simulink model "BD_SER_saber_cosim"  (Simulink 4.1.1)
settings: Solver=ode1  SolverMode=SingleTasking  StartTime=0.0  StopTime=max(cyc_mph(:,1))  FixedStep=1  MaxStep=1  RelTol=1e-3  AbsTol=1e-3
undefined symbols (not defined in the file): cs_fc_off2regen_pwr, cs_fc_spd_setpt_fun, cs_fc_trq_setpt_fun, cs_hi_soc, cs_lo_soc, cyc_mph, ess_max_volts_fun, ess_min_volts_fun, ess_on, ex_calc, fc_emis, fc_map_spd, fc_max_trq, fc_on, fc_spd_scale, fc_trq_scale, fd_ratio, gb_dnshift_load, gb_dnshift_spd, gb_gears_num, gb_num_init, gb_ratio, gb_shift_delay, gb_upshift_load, gb_upshift_spd, gc_map_spd, gc_max_trq, gc_spd_scale, gc_trq_scale, mc_map_spd, mc_max_trq, mc_spd_scale, mc_trq_scale, tc_gc_to_fc_ratio_fun, time_step, tx_speed_dep, vc_idle_bool, vc_idle_spd, wh_radius
libraries: lib_cosimulation x10, lib_outputs x8, lib_controls x5, lib_wheel x2, lib_help x2, lib_transmission x2, lib_accessory x2, lib_interactive x1, lib_drive_cycle x1, lib_exhaust x1, lib_fuel_converter x1, lib_vehicle x1
(part 1 of 2)
settings Model: LastModifiedBy=ssprik  SaveTime=off  SaveOutput=off  LimitDataPoints=off  UnconnectedLineMsg=none  RTWTemplateMakefile=grt_vc.tmf  ExtModeTrigMode=oneshot  ExtModeArmWhenConnect=off
settings Model: ModifiedComment=|
  | mokeefe -- Thu Apr 18 08:09:28 2002 -- Version 1.121
  | saving the model:
  | o "without the model browser open"
  | o with only top-level screen visible
  | o and with "fit to view" enabled
settings Model: ModifiedHistory=|
  | mokeefe -- Thu Apr 18 08:09:28 2002 -- Version 1.121
  | saving the model:
  | o "without the model browser open"
  | o with only top-level screen visible
  | o and with "fit to view" enabled

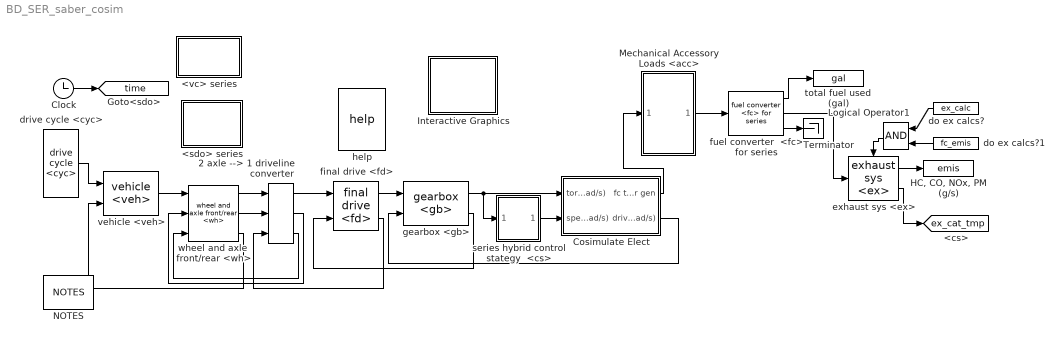
== system BD_SER_saber_cosim ==
  2 axle --> 1 driveline converter : lib_wheel/2 axle --> 1 driveline converter
      settings: RTWFcnNameOpts=Auto  RTWFileNameOpts=Auto
  <sdo> series : Subsystem
      settings: RTWFcnNameOpts=Auto  RTWFileNameOpts=Auto
      mask Display: image(imread('bdi_sdo.jpg'))
  <vc> series : Subsystem
      settings: RTWFcnNameOpts=Auto  RTWFileNameOpts=Auto
      mask Display: image(imread('bdi_vc.jpg'))
  Clock : Clock
      settings: DisplayTime=off  Decimation=10
  Cosimulate Elect : Subsystem  AncestorBlock=lib_cosimulation/SaberCosim
      settings: RTWFcnNameOpts=Auto  RTWFileNameOpts=Auto
      mask Display: image(imread('series_cosim.bmp'))
  "HC, CO, NOx, PM (g/s)" : ToWorkspace  VariableName=emis  SampleTime=0  SaveFormat=Array
  Interactive Graphics : Subsystem  BlockChoice=off
      link override off/Live Inputs/veh/roll res interactive: BlockChoice=roll res force req (N)
      settings: AttributesFormatString=%<BlockChoice>  TemplateBlock=lib_interactive/Interactive Graphics  MemberBlocks=off,on  RTWFcnNameOpts=Auto  RTWFileNameOpts=Auto
  Logical Operator1 : Logic  Orientation=left  Operator=AND  Inputs=2
  Mechanical Accessory Loads <acc> : Subsystem
      settings: RTWFcnNameOpts=Auto  RTWFileNameOpts=Auto
      mask Display: image(imread('bdi_acc_pic.bmp'))
  NOTES : lib_help/NOTES
  Terminator : Terminator
  do ex calcs? : Constant  Orientation=left  Value=ex_calc
  do ex calcs?1 : Constant  Orientation=left  Value=fc_emis
  drive cycle <cyc> : lib_drive_cycle/drive cycle <cyc>
  exhaust sys <ex> : lib_exhaust/exhaust sys <ex>
  final drive <fd> : lib_transmission/final drive <fd>
  fuel converter  <fc> for series : lib_fuel_converter/fuel converter  <fc> for series
      link override fuel use and EO emis Configurable Subsystem: BlockChoice=fuel use and EO emis
  gearbox <gb> : lib_transmission/gearbox <gb>
  help : lib_help/help
  series hybrid control stategy  <cs> : Subsystem
      settings: RTWFcnNameOpts=Auto  RTWFileNameOpts=Auto
      mask Display: image(imread('bdi_cs.jpg'))
  total fuel used  (gal) : ToWorkspace  VariableName=gal  SampleTime=0  SaveFormat=Array
  vehicle <veh> : lib_vehicle/vehicle <veh>
      link override config force req'd to overcome rolling resistance: BlockChoice=force req'd to overcome rolling resistance (N)
      link override config vehicle speed: BlockChoice=vehicle speed (m/s)
      link override rolling resistance force: BlockChoice=force req'd to overcome rolling resistance (N)
      link override vehicle speed: BlockChoice=vehicle speed (m/s)
  wheel and axle  front/rear <wh> : lib_wheel/wheel and axle  front//rear <wh>
  tag scope: ex_cat_tmp=global, time=global
  wires:
  gearbox <gb>/1 -> Cosimulate Elect/1(torque and speed req'd at input side of gearbox (Nm),(rad/s)), series hybrid control stategy  <cs>/1(gb trq & spd r)
  gearbox <gb>/2 -> final drive <fd>/2
  final drive <fd>/1 -> gearbox <gb>/1
  drive cycle <cyc>/1 -> vehicle <veh>/1
  Clock/1 -> [time]
  fuel converter  <fc> for series/2 -> exhaust sys <ex>/1
  fuel converter  <fc> for series/1 -> total fuel used  (gal)/1
  Logical Operator1/1 -> exhaust sys <ex>/Enable
  do ex calcs?/1 -> Logical Operator1/1
  exhaust sys <ex>/1 -> "HC, CO, NOx, PM (g/s)"/1
  do ex calcs?1/1 -> Logical Operator1/2
  exhaust sys <ex>/2 -> [ex_cat_tmp]
  Cosimulate Elect/2("drive torque and speed avail. at rotor (Nm), (rad/s)") -> gearbox <gb>/2
  series hybrid control stategy  <cs>/1(engine speed and torque (Nm) (rad/s)) -> Cosimulate Elect/2(speed and torque  avail from fc  (Nm) (rad/s))
  fuel converter  <fc> for series/3 -> Terminator/1
  Cosimulate Elect/1(fc trq and spd req'd for gen) -> Mechanical Accessory Loads <acc>/1(trq and spd)
  Mechanical Accessory Loads <acc>/1(trq and spd1) -> fuel converter  <fc> for series/1
  wheel and axle  front/rear <wh>/1 -> 2 axle --> 1 driveline converter/1
  wheel and axle  front/rear <wh>/2 -> 2 axle --> 1 driveline converter/2
  2 axle --> 1 driveline converter/1 -> final drive <fd>/1
  2 axle --> 1 driveline converter/2 -> wheel and axle  front/rear <wh>/2
  2 axle --> 1 driveline converter/3 -> wheel and axle  front/rear <wh>/3
  vehicle <veh>/1 -> wheel and axle  front/rear <wh>/1
  final drive <fd>/2 -> 2 axle --> 1 driveline converter/3
  wheel and axle  front/rear <wh>/3 -> vehicle <veh>/2

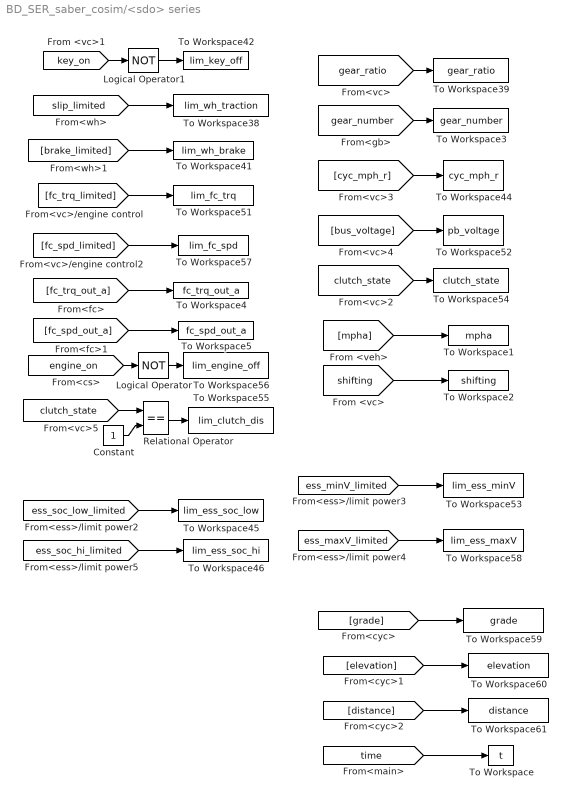
== system BD_SER_saber_cosim/<sdo> series ==
  Constant : Constant  Value=1
  Logical Operator : Logic  Operator=NOT  Inputs=1
  Logical Operator1 : Logic  Operator=NOT  Inputs=1
  Relational Operator : RelationalOperator  Operator===
  To Workspace : ToWorkspace  VariableName=t  SampleTime=0  SaveFormat=Array
  To Workspace1 : ToWorkspace  VariableName=mpha  SampleTime=-1  SaveFormat=Array
  To Workspace2 : ToWorkspace  VariableName=shifting  SampleTime=-1  SaveFormat=Array
  To Workspace3 : ToWorkspace  VariableName=gear_number  SampleTime=-1  SaveFormat=Array
  To Workspace38 : ToWorkspace  VariableName=lim_wh_traction  SampleTime=-1  SaveFormat=Array
  To Workspace39 : ToWorkspace  VariableName=gear_ratio  SampleTime=-1  SaveFormat=Array
  To Workspace4 : ToWorkspace  VariableName=fc_trq_out_a  SampleTime=-1  SaveFormat=Array
  To Workspace41 : ToWorkspace  VariableName=lim_wh_brake  SampleTime=-1  SaveFormat=Array
  To Workspace42 : ToWorkspace  VariableName=lim_key_off  SampleTime=-1  SaveFormat=Array
  To Workspace44 : ToWorkspace  VariableName=cyc_mph_r  SampleTime=-1  SaveFormat=Array
  To Workspace45 : ToWorkspace  VariableName=lim_ess_soc_low  SampleTime=-1  SaveFormat=Array
  To Workspace46 : ToWorkspace  VariableName=lim_ess_soc_hi  SampleTime=-1  SaveFormat=Array
  To Workspace5 : ToWorkspace  VariableName=fc_spd_out_a  SampleTime=-1  SaveFormat=Array
  To Workspace51 : ToWorkspace  VariableName=lim_fc_trq  SampleTime=-1  SaveFormat=Array
  To Workspace52 : ToWorkspace  VariableName=pb_voltage  SampleTime=-1  SaveFormat=Array
  To Workspace53 : ToWorkspace  VariableName=lim_ess_minV  SampleTime=-1  SaveFormat=Array
  To Workspace54 : ToWorkspace  VariableName=clutch_state  SampleTime=-1  SaveFormat=Array
  To Workspace55 : ToWorkspace  VariableName=lim_clutch_dis  SampleTime=-1  SaveFormat=Array
  To Workspace56 : ToWorkspace  VariableName=lim_engine_off  SampleTime=-1  SaveFormat=Array
  To Workspace57 : ToWorkspace  VariableName=lim_fc_spd  SampleTime=-1  SaveFormat=Array
  To Workspace58 : ToWorkspace  VariableName=lim_ess_maxV  SampleTime=-1  SaveFormat=Array
  To Workspace59 : ToWorkspace  VariableName=grade  SampleTime=-1  SaveFormat=Array
  To Workspace60 : ToWorkspace  VariableName=elevation  SampleTime=-1  SaveFormat=Array
  To Workspace61 : ToWorkspace  VariableName=distance  SampleTime=-1  SaveFormat=Array
  wires:
  [time] -> To Workspace/1
  [clutch_state] -> Relational Operator/1
  [fc_spd_out_a] -> To Workspace5/1
  [fc_trq_out_a] -> To Workspace4/1
  [ess_soc_hi_limited] -> To Workspace46/1
  [ess_soc_low_limited] -> To Workspace45/1
  Logical Operator/1 -> To Workspace56/1
  [engine_on] -> Logical Operator/1
  Constant/1 -> Relational Operator/2
  Relational Operator/1 -> To Workspace55/1
  [distance] -> To Workspace61/1
  [elevation] -> To Workspace60/1
  [grade] -> To Workspace59/1
  [ess_minV_limited] -> To Workspace53/1
  [ess_maxV_limited] -> To Workspace58/1
  Logical Operator1/1 -> To Workspace42/1
  [key_on] -> Logical Operator1/1
  [shifting] -> To Workspace2/1
  [mpha] -> To Workspace1/1
  [clutch_state] -> To Workspace54/1
  [bus_voltage] -> To Workspace52/1
  [cyc_mph_r] -> To Workspace44/1
  [gear_ratio] -> To Workspace39/1
  [slip_limited] -> To Workspace38/1
  [brake_limited] -> To Workspace41/1
  [fc_spd_limited] -> To Workspace57/1
  [fc_trq_limited] -> To Workspace51/1
  [gear_number] -> To Workspace3/1

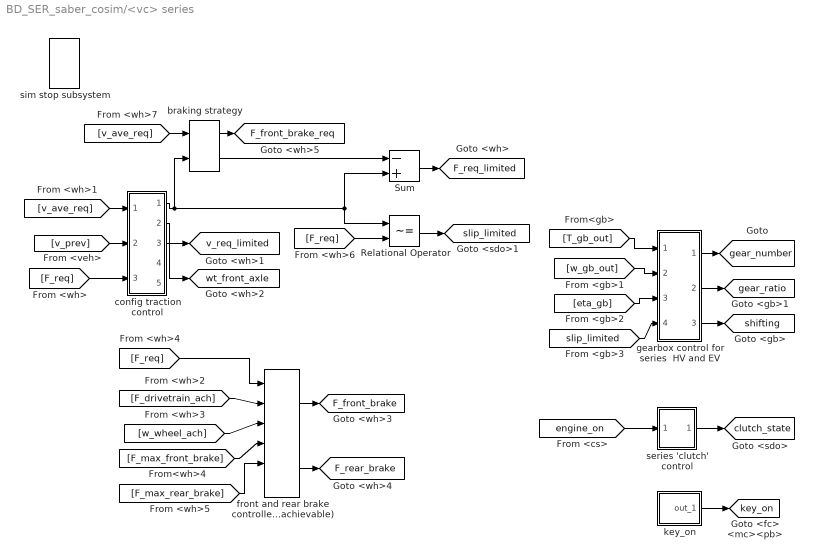
== system BD_SER_saber_cosim/<vc> series ==
  Relational Operator : RelationalOperator  Operator=~=
  Sum : Sum  Inputs=-+  SaturateOnIntegerOverflow=on
  braking strategy : lib_controls/SubSystem/braking strategy
      settings: RTWFcnNameOpts=Auto  RTWFileNameOpts=Auto
  config traction control : Subsystem  BlockChoice=traction control 2 axle
      settings: AttributesFormatString=%<BlockChoice>  TemplateBlock=lib_controls/SubSystem/config traction control  MemberBlocks=traction control 2 axle,traction control J2452 2 axle  RTWFcnNameOpts=Auto  RTWFileNameOpts=Auto
  front and rear brake controller (achievable) : lib_controls/SubSystem/front and rear brake controller (achievable)
      settings: RTWFcnNameOpts=Auto  RTWFileNameOpts=Auto
  gearbox control for series  HV and EV : Subsystem
      settings: RTWFcnNameOpts=Auto  RTWFileNameOpts=Auto
  key_on : Subsystem  mask(Repeating table){@1=vc_key_on(:,1), @2=vc_key_on(:,2)}
      mask prompts: @1 "Time values:"; @2 "Output values:"
      mask help:
      | Repeating table.
      | Enter values of time and output for first cycle.
      mask init:
      | period = max(@1); t = @1; y = @2;
      settings: RTWFcnNameOpts=Auto  RTWFileNameOpts=Auto
      mask Help: Repeats cycle given in table. Time values should be monotonically increasing.
  series 'clutch' control : Subsystem
      settings: RTWFcnNameOpts=Auto  RTWFileNameOpts=Auto
  sim stop subsystem : lib_controls/SubSystem/sim stop subsystem
      settings: RTWFcnNameOpts=Auto  RTWFileNameOpts=Auto
  tag scope: F_front_brake=global, F_front_brake_req=global, F_rear_brake=global, F_req_limited=global, clutch_state=global, gear_number=global, gear_ratio=global, key_on=global, shifting=global, slip_limited=global, v_req_limited=global, wt_front_axle=global
  wires:
  gearbox control for series  HV and EV/1("gear number, out") -> [gear_number]
  gearbox control for series  HV and EV/2("gear ratio, out") -> [gear_ratio]
  gearbox control for series  HV and EV/3("shifting, out") -> [shifting]
  [v_ave_req] -> config traction control/1(time-average vehicle speed  req'd (m/s))
  [F_req] -> Relational Operator/2
  Relational Operator/1 -> [slip_limited]
  Sum/1 -> [F_req_limited]
  [F_req] -> config traction control/3(total tractive force req'd (N))
  config traction control/3(weight on front axle (N)) -> [wt_front_axle]
  config traction control/2(req'd speed (m/s)) -> [v_req_limited]
  [v_prev] -> config traction control/2(vehicle speed at beginning of time  step (m/s))
  config traction control/1(req'd force (N)) -> Relational Operator/1, Sum/2, braking strategy/2
  braking strategy/2 -> Sum/1
  [v_ave_req] -> braking strategy/1
  braking strategy/1 -> [F_front_brake_req]
  [F_req] -> front and rear brake controller (achievable)/1
  front and rear brake controller (achievable)/2 -> [F_rear_brake]
  [F_max_rear_brake] -> front and rear brake controller (achievable)/5
  [F_max_front_brake] -> front and rear brake controller (achievable)/4
  [w_wheel_ach] -> front and rear brake controller (achievable)/3
  [F_drivetrain_ach] -> front and rear brake controller (achievable)/2
  front and rear brake controller (achievable)/1 -> [F_front_brake]
  key_on/1(out_1) -> [key_on]
  [engine_on] -> series 'clutch' control/1(engine on)
  series 'clutch' control/1(clutch state) -> [clutch_state]
  [slip_limited] -> gearbox control for series  HV and EV/4(tires are at traction limit)
  [T_gb_out] -> gearbox control for series  HV and EV/1(gb_trq_out_r)
  [w_gb_out] -> gearbox control for series  HV and EV/2(gb_spd_out_r)
  [eta_gb] -> gearbox control for series  HV and EV/3(prev. Pout/Pin)

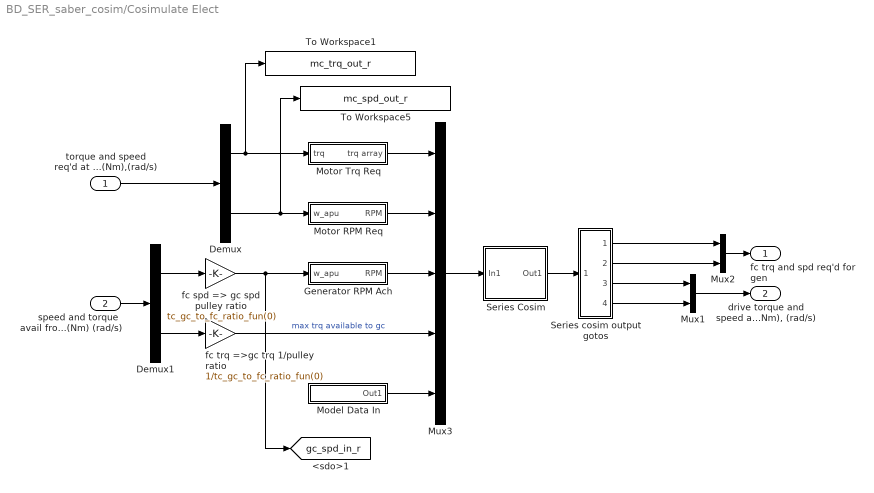
== system BD_SER_saber_cosim/Cosimulate Elect ==
  torque and speed req'd at input side of gearbox (Nm),(rad/s) : Inport  Port=1  LatchInput=off
  speed and torque  avail from fc  (Nm) (rad/s) : Inport  Port=2  LatchInput=off  PortDimensions=2
  Demux : Demux  Outputs=2  BusSelectionMode=off
  Demux1 : Demux  Outputs=2  BusSelectionMode=off
  Generator RPM Ach : Subsystem
      settings: RTWFcnNameOpts=Auto  RTWFileNameOpts=Auto
  Model Data In : Subsystem
      settings: RTWFcnNameOpts=Auto  RTWFileNameOpts=Auto
      mask Display: disp('Series')
  Motor RPM Req : Subsystem
      settings: RTWFcnNameOpts=Auto  RTWFileNameOpts=Auto
  Motor Trq Req : Subsystem
      settings: RTWFcnNameOpts=Auto  RTWFileNameOpts=Auto
  Mux1 : Mux  Inputs=2
  Mux2 : Mux  Inputs=2
  Mux3 : Mux  Inputs=5
  Series Cosim : Subsystem  BlockChoice=Saber Text File Exchange
      settings: AttributesFormatString=%<BlockChoice>  TemplateBlock=lib_cosimulation/Series Cosim  MemberBlocks=Saber Text File Exchange,Series Saber Cosim,Series Simplorer Cosim  RTWFcnNameOpts=Auto  RTWFileNameOpts=Auto
  Series cosim output gotos : Subsystem
      settings: RTWFcnNameOpts=Auto  RTWFileNameOpts=Auto
  To Workspace1 : ToWorkspace  VariableName=mc_trq_out_r  SampleTime=-1  SaveFormat=Array
  To Workspace5 : ToWorkspace  VariableName=mc_spd_out_r  SampleTime=-1  SaveFormat=Array
  fc spd => gc spd pulley ratio : Gain  Gain=tc_gc_to_fc_ratio_fun(0)  Multiplication=Element-wise(K.*u)  SaturateOnIntegerOverflow=on
  fc trq =>gc trq 1/pulley ratio : Gain  Gain=1/tc_gc_to_fc_ratio_fun(0)  Multiplication=Element-wise(K.*u)  SaturateOnIntegerOverflow=on
  fc trq and spd req'd for gen : Outport  Port=1
  "drive torque and speed avail. at rotor (Nm), (rad/s)" : Outport  Port=2  InitialOutput=0
  tag scope: gc_spd_in_r=global
  wires:
  torque and speed req'd at input side of gearbox (Nm),(rad/s)/1 -> Demux/1
  Mux3/1 -> Series Cosim/1(In1)
  Series Cosim/1(Out1) -> Series cosim output gotos/1(In1)
  Mux1/1 -> "drive torque and speed avail. at rotor (Nm), (rad/s)"/1
  Series cosim output gotos/1(fc_trq_r) -> Mux2/1
  Demux/2 -> Motor RPM Req/1(w_apu), To Workspace5/1
  Motor RPM Req/1(RPM) -> Mux3/2
  Demux/1 -> Motor Trq Req/1(trq), To Workspace1/1
  Motor Trq Req/1(trq array) -> Mux3/1
  Series cosim output gotos/4(mc_spd) -> Mux1/2
  Series cosim output gotos/3(mc_trq) -> Mux1/1
  Series cosim output gotos/2(fc_spd_r) -> Mux2/2
  Mux2/1 -> fc trq and spd req'd for gen/1
  Generator RPM Ach/1(RPM) -> Mux3/3
  fc spd => gc spd pulley ratio/1 -> Generator RPM Ach/1(w_apu), [gc_spd_in_r]
  Model Data In/1(Out1) -> Mux3/5
  Demux1/1 -> fc spd => gc spd pulley ratio/1
  Demux1/2 -> fc trq =>gc trq 1/pulley ratio/1
  speed and torque  avail from fc  (Nm) (rad/s)/1 -> Demux1/1
  fc trq =>gc trq 1/pulley ratio/1 -> Mux3/4  "max trq available to gc"

== system BD_SER_saber_cosim/Interactive Graphics ==
  off : lib_interactive/off  Tag=Altia_off  Orientation=up

== system BD_SER_saber_cosim/Mechanical Accessory Loads <acc> ==
  trq and spd : Inport  Port=1  LatchInput=off
  Demux2 : Demux  Outputs=2  BusSelectionMode=off
  Mux2 : Mux  Inputs=2
  Sum : Sum  Inputs=++  SaturateOnIntegerOverflow=on
  trq and spd1 : Outport  Port=1
  wires:
  Mux2/1 -> trq and spd1/1
  trq and spd/1 -> Demux2/1
  Sum/1 -> Mux2/1
  [acc_total_mech_trq] -> Sum/1
  Demux2/1 -> Sum/2
  Demux2/2 -> Mux2/2

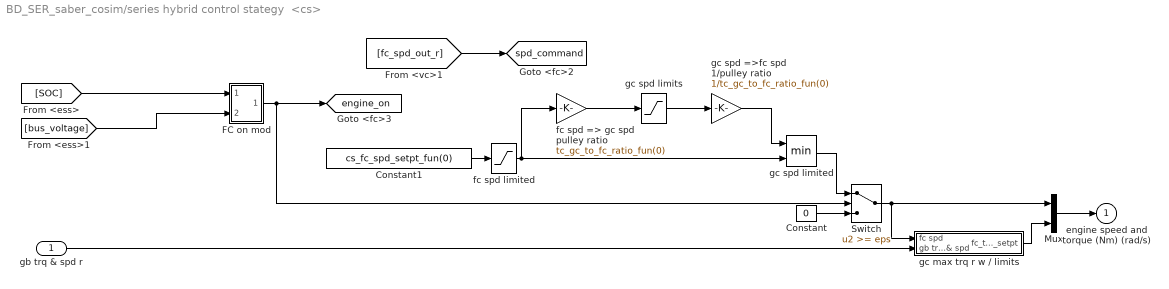
== system BD_SER_saber_cosim/series hybrid control stategy  <cs> ==
  gb trq & spd r : Inport  Port=1  LatchInput=off
  Constant : Constant  Value=0
  Constant1 : Constant  Value=cs_fc_spd_setpt_fun(0)
  FC on mod : Subsystem
      settings: RTWFcnNameOpts=Auto  RTWFileNameOpts=Auto
  Mux : Mux  Inputs=2
  Switch : Switch  Threshold=eps
  fc spd limited : Saturate  UpperLimit=max(fc_map_spd)*fc_spd_scale  LowerLimit=0  LinearizeAsGain=on
  fc spd => gc spd pulley ratio : Gain  Gain=tc_gc_to_fc_ratio_fun(0)  Multiplication=Element-wise(K.*u)  SaturateOnIntegerOverflow=on
  gc max trq r w / limits : Subsystem
      settings: RTWFcnNameOpts=Auto  RTWFileNameOpts=Auto
  gc spd limited : MinMax  Function=min  Inputs=2
  gc spd limits : Saturate  UpperLimit=max(gc_map_spd)*gc_spd_scale  LowerLimit=0  LinearizeAsGain=on
  gc spd =>fc spd 1/pulley ratio : Gain  Gain=1/tc_gc_to_fc_ratio_fun(0)  Multiplication=Element-wise(K.*u)  SaturateOnIntegerOverflow=on
  engine speed and torque (Nm) (rad/s) : Outport  Port=1  InitialOutput=0
  tag scope: engine_on=global, spd_command=global
  wires:
  FC on mod/1(FC on) -> Switch/2, [engine_on]
  [fc_spd_out_r] -> [spd_command]
  Constant/1 -> Switch/3
  gb trq & spd r/1 -> gc max trq r w / limits/2(gb trq & spd)
  [bus_voltage] -> FC on mod/2(bus voltage)
  [SOC] -> FC on mod/1(SOC)
  Constant1/1 -> fc spd limited/1
  fc spd limited/1 -> gc spd limited/2, fc spd => gc spd pulley ratio/1
  Mux/1 -> engine speed and torque (Nm) (rad/s)/1
  Switch/1 -> gc max trq r w / limits/1(fc spd), Mux/1
  gc max trq r w / limits/1(fc_trq_setpt) -> Mux/2
  gc spd limited/1 -> Switch/1
  fc spd => gc spd pulley ratio/1 -> gc spd limits/1
  gc spd =>fc spd 1/pulley ratio/1 -> gc spd limited/1
  gc spd limits/1 -> gc spd =>fc spd 1/pulley ratio/1

== system BD_SER_saber_cosim/<vc> series/config traction control ==
  time-average vehicle speed  req'd (m/s) : Inport  Port=1  LatchInput=off
  vehicle speed at beginning of time  step (m/s) : Inport  Port=2  LatchInput=off
  total tractive force req'd (N) : Inport  Port=3  LatchInput=off
  traction control 2 axle : lib_controls/SubSystem/traction control 2 axle
      settings: RTWFcnNameOpts=Auto  RTWFileNameOpts=Auto
  req'd force (N) : Outport  Port=1
  req'd speed (m/s) : Outport  Port=2
  weight on front axle (N) : Outport  Port=3
  weight on rear axle (N) : Outport  Port=4
  front/total  traction ratio : Outport  Port=5
  wires:
  time-average vehicle speed  req'd (m/s)/1 -> traction control 2 axle/1
  vehicle speed at beginning of time  step (m/s)/1 -> traction control 2 axle/2
  total tractive force req'd (N)/1 -> traction control 2 axle/3
  traction control 2 axle/1 -> req'd force (N)/1
  traction control 2 axle/2 -> req'd speed (m/s)/1
  traction control 2 axle/3 -> weight on front axle (N)/1
  traction control 2 axle/4 -> weight on rear axle (N)/1
  traction control 2 axle/5 -> front/total  traction ratio/1

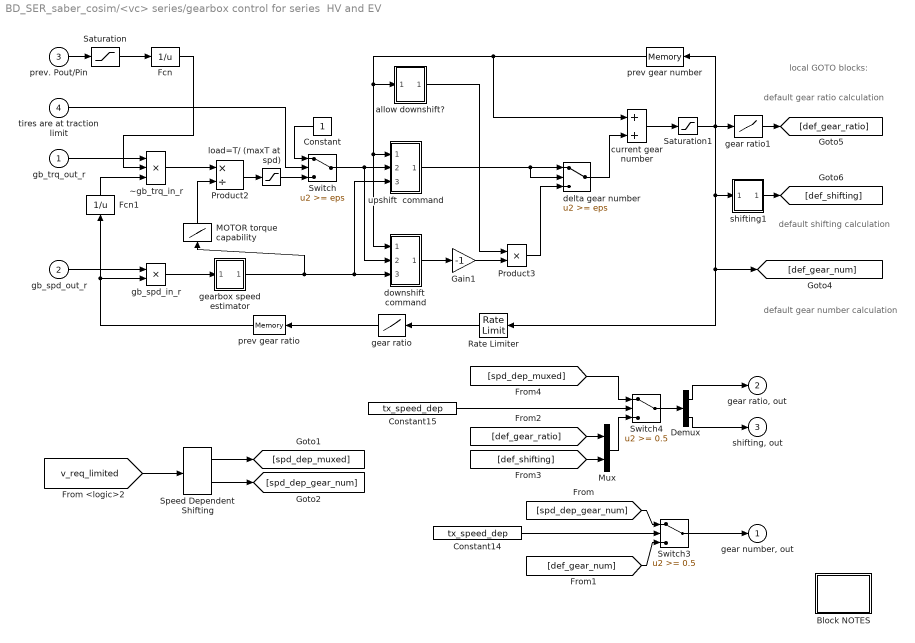
== system BD_SER_saber_cosim/<vc> series/gearbox control for series  HV and EV ==
  note: local GOTO blocks:
  note: default gear ratio
      | calculation
  note: default shifting
      | calculation
  note: default gear number
      | calculation
  gb_trq_out_r : Inport  Port=1  LatchInput=off
  gb_spd_out_r : Inport  Port=2  LatchInput=off
  prev. Pout/Pin : Inport  Port=3  LatchInput=off
  tires are at traction limit : Inport  Port=4  LatchInput=off
  Block NOTES : Subsystem
      settings: RTWFcnNameOpts=Auto  RTWFileNameOpts=Auto
      mask Display: disp('Block\nNOTES')
  Constant : Constant  Orientation=left  Value=1
  Constant14 : Constant  Value=tx_speed_dep
  Constant15 : Constant  Value=tx_speed_dep
  Demux : Demux  Outputs=2  BusSelectionMode=off
  Fcn : Fcn  Expr=1/u
  Fcn1 : Fcn  Orientation=up  Expr=1/u
  Gain1 : Gain  Gain=-1  Multiplication=Element-wise(K.*u)  SaturateOnIntegerOverflow=on
  MOTOR torque capability : Lookup  Orientation=up  InputValues=mc_map_spd*mc_spd_scale  OutputValues=mc_max_trq*mc_trq_scale+eps
  Mux : Mux  Inputs=2
  Product2 : Product  Inputs=*/  Multiplication=Element-wise(.*)  SaturateOnIntegerOverflow=on
  Product3 : Product  Inputs=2  Multiplication=Element-wise(.*)  SaturateOnIntegerOverflow=on
  Rate Limiter : RateLimiter  Orientation=left  RisingSlewLimit=1/(gb_shift_delay+eps)  FallingSlewLimit=-1/(gb_shift_delay+eps)
  Saturation : Saturate  UpperLimit=1  LowerLimit=0.2  LinearizeAsGain=on
  Saturation1 : Saturate  UpperLimit=gb_gears_num  LowerLimit=1  LinearizeAsGain=on
  Speed Dependent Shifting : lib_controls/SubSystem/Speed Dependent Shifting
      settings: RTWFcnNameOpts=Auto  RTWFileNameOpts=Auto
  Switch : Switch  Threshold=eps
  Switch3 : Switch  Threshold=0.5
  Switch4 : Switch  Threshold=0.5
  allow downshift? : Subsystem
      settings: RTWFcnNameOpts=Auto  RTWFileNameOpts=Auto
  current gear number : Sum  Inputs=++  SaturateOnIntegerOverflow=on
  delta gear number : Switch  Threshold=eps
  downshift  command : Subsystem
      settings: RTWFcnNameOpts=Auto  RTWFileNameOpts=Auto
  gb_spd_in_r : Product  Inputs=2  Multiplication=Element-wise(.*)  SaturateOnIntegerOverflow=on
  gear ratio : Lookup  Orientation=left  InputValues=[1:length(gb_ratio)]  OutputValues=gb_ratio
  gear ratio1 : Lookup  InputValues=[1:length(gb_ratio)]  OutputValues=gb_ratio
  gearbox speed estimator : Subsystem
      settings: RTWFcnNameOpts=Auto  RTWFileNameOpts=Auto
  load=T/ (maxT at spd) : Saturate  UpperLimit=1  LowerLimit=0  LinearizeAsGain=on
  prev gear number : Memory  Orientation=left  X0=1  InheritSampleTime=off
      settings: RTWStateStorageClass=Auto
  prev gear ratio : Memory  Orientation=left  X0=gb_ratio(1)  InheritSampleTime=off
      settings: RTWStateStorageClass=Auto
  shifting1 : Subsystem
      settings: RTWFcnNameOpts=Auto  RTWFileNameOpts=Auto
  upshift  command : Subsystem
      settings: RTWFcnNameOpts=Auto  RTWFileNameOpts=Auto
  ~gb_trq_in_r : Product  Inputs=3  Multiplication=Element-wise(.*)  SaturateOnIntegerOverflow=on
  "gear number, out" : Outport  Port=1  InitialOutput=0
  "gear ratio, out" : Outport  Port=2  InitialOutput=0
  "shifting, out" : Outport  Port=3  InitialOutput=0
  wires:
  shifting1/1(out_1) -> [def_shifting]
  gear ratio1/1 -> [def_gear_ratio]
  Switch3/1 -> "gear number, out"/1
  Demux/2 -> "shifting, out"/1
  Demux/1 -> "gear ratio, out"/1
  Speed Dependent Shifting/2 -> [spd_dep_gear_num]
  Speed Dependent Shifting/1 -> [spd_dep_muxed]
  [v_req_limited] -> Speed Dependent Shifting/1
  [spd_dep_gear_num] -> Switch3/1
  Switch4/1 -> Demux/1
  [def_shifting] -> Mux/2
  [def_gear_ratio] -> Mux/1
  Mux/1 -> Switch4/3
  [spd_dep_muxed] -> Switch4/1
  Constant15/1 -> Switch4/2
  [def_gear_num] -> Switch3/3
  Constant14/1 -> Switch3/2
  prev gear number/1 -> current gear number/1, downshift  command/1(prev gear number), upshift  command/1(prev gear number), allow downshift?/1(prev gearnum)
  Saturation1/1 -> [def_gear_num], Rate Limiter/1, shifting1/1(gear number), gear ratio1/1, prev gear number/1
  Switch/1 -> downshift  command/2(engine load), upshift  command/2(engine load)
  Constant/1 -> Switch/1
  tires are at traction limit/1 -> Switch/2
  load=T/ (maxT at spd)/1 -> Switch/3
  Fcn/1 -> ~gb_trq_in_r/2
  ~gb_trq_in_r/1 -> Product2/1
  Product2/1 -> load=T/ (maxT at spd)/1
  MOTOR torque capability/1 -> Product2/2
  Fcn1/1 -> ~gb_trq_in_r/3
  delta gear number/1 -> current gear number/2
  prev gear ratio/1 -> gb_spd_in_r/2, Fcn1/1
  allow downshift?/1(allow shift) -> Product3/1
  Product3/1 -> delta gear number/3
  Gain1/1 -> Product3/2
  downshift  command/1(command) -> Gain1/1
  gb_spd_out_r/1 -> gb_spd_in_r/1
  Rate Limiter/1 -> gear ratio/1
  gear ratio/1 -> prev gear ratio/1
  upshift  command/1(command) -> delta gear number/2, delta gear number/1
  gb_trq_out_r/1 -> ~gb_trq_in_r/1
  prev. Pout/Pin/1 -> Saturation/1
  Saturation/1 -> Fcn/1
  current gear number/1 -> Saturation1/1
  gb_spd_in_r/1 -> gearbox speed estimator/1(gb_spd_in_r if no gear change)
  gearbox speed estimator/1(Out1) -> upshift  command/3(engine speed), downshift  command/3(engine speed), MOTOR torque capability/1

== system BD_SER_saber_cosim/<vc> series/key_on ==
  Clock : Clock
      settings: DisplayTime=off  Decimation=10
  Fcn1 : Fcn  Expr=rem(u[1],period)
  Look-Up Table : Lookup  InputValues=t  OutputValues=y
  out_1 : Outport  Port=1  InitialOutput=0
  wires:
  Fcn1/1 -> Look-Up Table/1
  Clock/1 -> Fcn1/1
  Look-Up Table/1 -> out_1/1

== system BD_SER_saber_cosim/<vc> series/series 'clutch' control ==
  engine on : Inport  Port=1  LatchInput=off
  Block NOTES : Subsystem
      settings: RTWFcnNameOpts=Auto  RTWFileNameOpts=Auto
      mask Display: disp('Block\nNOTES')
  Clock : Clock
      settings: DisplayTime=off  Decimation=10
  Constant6 : Constant  Orientation=left  Value=1
  Constant7 : Constant  Orientation=left  Value=3
  Memory1 : Memory  X0=cyc_mph(1,2)>0  InheritSampleTime=off
      settings: RTWStateStorageClass=Auto
  Memory2 : Memory  X0=-1  InheritSampleTime=off
      settings: RTWStateStorageClass=Auto
  Sum : Sum  Inputs=+-  SaturateOnIntegerOverflow=on
  Switch : Switch  Threshold=eps
  Switch1 : Switch  Threshold=0.5
  Transport Delay : TransportDelay  DelayTime=0.5  InitialInput=0  BufferSize=1024  PadeOrder=0
  clutch slipping1 : Logic  Operator=AND  Inputs=2
  clutch slipping2 : Logic  Operator=AND  Inputs=2
  clutch state : Outport  Port=1
  wires:
  Memory1/1 -> clutch slipping1/2
  Constant7/1 -> Switch/1
  Switch1/1 -> Switch/2
  Switch/1 -> clutch state/1
  Constant6/1 -> Switch/3
  clutch slipping1/1 -> Switch1/1
  Transport Delay/1 -> clutch slipping2/2
  clutch slipping2/1 -> Switch1/3
  Clock/1 -> Sum/1, Memory2/1
  Memory2/1 -> Sum/2
  Sum/1 -> Switch1/2
  engine on/1 -> clutch slipping1/1, Memory1/1, Transport Delay/1, clutch slipping2/1

== system BD_SER_saber_cosim/Cosimulate Elect/Generator RPM Ach ==
  w_apu : Inport  Port=1  LatchInput=off
  Constant : Constant  Value=0
  Enabled Subsystem : Subsystem  TreatAsAtomicUnit=on
      settings: RTWFcnNameOpts=Auto  RTWFileNameOpts=Auto
  IC : InitialCondition  Value=time_step
  Memory1 : Memory  X0=.001  InheritSampleTime=on
      settings: RTWStateStorageClass=Auto
  Memory2 : Memory  X0=80  InheritSampleTime=on
      settings: RTWStateStorageClass=Auto
  Mux3 : Mux  Inputs=6
  Relational Operator : RelationalOperator  Operator===
  Saturation : Saturate  UpperLimit=inf  LowerLimit=.001  LinearizeAsGain=on
  "rad/s -> rpm1" : Gain  Gain=60/(2*pi)  Multiplication=Element-wise(K.*u)  SaturateOnIntegerOverflow=on
  RPM : Outport  Port=1
  wires:
  Relational Operator/1 -> Enabled Subsystem/Enable
  [time] -> Relational Operator/2
  Enabled Subsystem/1(Out1) -> Mux3/2
  Memory2/1 -> Mux3/4
  Mux3/1 -> RPM/1
  IC/1 -> Mux3/5
  Saturation/1 -> Memory1/1
  [time] -> Saturation/1
  Memory1/1 -> Mux3/3
  [time] -> IC/1
  Constant/1 -> Relational Operator/1, Mux3/1
  w_apu/1 -> "rad/s -> rpm1"/1  "w_apu"
  "rad/s -> rpm1"/1 -> Memory2/1, Mux3/6, Enabled Subsystem/1(In1)

== system BD_SER_saber_cosim/Cosimulate Elect/Model Data In ==
  Aux Loads 14V and 42V : Subsystem
      settings: RTWFcnNameOpts=Auto  RTWFileNameOpts=Auto
  DC/DC converter : lib_cosimulation/DC//DC converter
      settings: RTWFcnNameOpts=Auto  RTWFileNameOpts=Auto
  Generator reg : lib_cosimulation/Generator reg
      settings: RTWFcnNameOpts=Auto  RTWFileNameOpts=Auto
  Mux : Mux  Inputs=7
  Regulator : lib_cosimulation/Regulator
      settings: RTWFcnNameOpts=Auto  RTWFileNameOpts=Auto
  ess param inputs : Subsystem  BlockChoice=Rint
      settings: AttributesFormatString=%<BlockChoice>  TemplateBlock=lib_cosimulation/ess param inputs  MemberBlocks=Rint,Saber lib pb  RTWFcnNameOpts=Auto  RTWFileNameOpts=Auto
  ess2 param inputs : Subsystem  BlockChoice=Saber lib pb2
      settings: AttributesFormatString=%<BlockChoice>  TemplateBlock=lib_cosimulation/ess2 param inputs  MemberBlocks=Rint2,Saber lib pb2  RTWFcnNameOpts=Auto  RTWFileNameOpts=Auto
  motor : lib_cosimulation/motor
      settings: RTWFcnNameOpts=Auto  RTWFileNameOpts=Auto
  Out1 : Outport  Port=1
  wires:
  DC/DC converter/1 -> Mux/2
  Aux Loads 14V and 42V/1(Out1) -> Mux/1
  Mux/1 -> Out1/1
  Regulator/1 -> Mux/3
  ess param inputs/1(Out1) -> Mux/4
  ess2 param inputs/1(Out1) -> Mux/5
  Generator reg/1 -> Mux/6
  motor/1 -> Mux/7

== system BD_SER_saber_cosim/Cosimulate Elect/Motor RPM Req ==
  w_apu : Inport  Port=1  LatchInput=off
  Constant : Constant  Value=0
  Enabled Subsystem : Subsystem  TreatAsAtomicUnit=on
      settings: RTWFcnNameOpts=Auto  RTWFileNameOpts=Auto
  IC : InitialCondition  Value=time_step
  Memory1 : Memory  X0=.001  InheritSampleTime=on
      settings: RTWStateStorageClass=Auto
  Memory2 : Memory  X0=0  InheritSampleTime=on
      settings: RTWStateStorageClass=Auto
  Mux3 : Mux  Inputs=[1 1 1 1 1 1]
  Relational Operator : RelationalOperator  Operator===
  Saturation : Saturate  UpperLimit=inf  LowerLimit=.001  LinearizeAsGain=on
  "rad/s -> rpm1" : Gain  Gain=60/(2*pi)  Multiplication=Element-wise(K.*u)  SaturateOnIntegerOverflow=on
  RPM : Outport  Port=1
  wires:
  Relational Operator/1 -> Enabled Subsystem/Enable
  [time] -> Relational Operator/2
  Enabled Subsystem/1(Out1) -> Mux3/2
  Memory2/1 -> Mux3/4
  Mux3/1 -> RPM/1
  IC/1 -> Mux3/5
  Saturation/1 -> Memory1/1
  [time] -> Saturation/1
  Memory1/1 -> Mux3/3
  [time] -> IC/1
  Constant/1 -> Relational Operator/1, Mux3/1
  w_apu/1 -> "rad/s -> rpm1"/1
  "rad/s -> rpm1"/1 -> Memory2/1, Mux3/6, Enabled Subsystem/1(In1)

== system BD_SER_saber_cosim/Cosimulate Elect/Motor Trq Req ==
  trq : Inport  Port=1  LatchInput=off
  Constant : Constant  Value=0
  Enabled Subsystem : Subsystem  TreatAsAtomicUnit=on
      settings: RTWFcnNameOpts=Auto  RTWFileNameOpts=Auto
  IC : InitialCondition  Value=time_step
  Memory1 : Memory  X0=.001  InheritSampleTime=on
      settings: RTWStateStorageClass=Auto
  Memory2 : Memory  X0=0  InheritSampleTime=on
      settings: RTWStateStorageClass=Auto
  Mux3 : Mux  Inputs=[1 1 1 1 1 1]
  Relational Operator : RelationalOperator  Operator===
  Saturation : Saturate  UpperLimit=inf  LowerLimit=.001  LinearizeAsGain=on
  trq array : Outport  Port=1
  wires:
  trq/1 -> Memory2/1, Mux3/6, Enabled Subsystem/1(In1)
  Constant/1 -> Relational Operator/1, Mux3/1
  [time] -> IC/1
  Memory1/1 -> Mux3/3
  [time] -> Saturation/1
  Saturation/1 -> Memory1/1
  IC/1 -> Mux3/5
  Mux3/1 -> trq array/1
  Memory2/1 -> Mux3/4
  Enabled Subsystem/1(Out1) -> Mux3/2
  [time] -> Relational Operator/2
  Relational Operator/1 -> Enabled Subsystem/Enable

== system BD_SER_saber_cosim/Cosimulate Elect/Series Cosim ==
  In1 : Inport  Port=1  LatchInput=off
  Saber Text File Exchange : lib_cosimulation/Saber Text File Exchange  AncestorBlock=lib_cosimulation/SaberCosim
  Out1 : Outport  Port=1
  wires:
  In1/1 -> Saber Text File Exchange/1
  Saber Text File Exchange/1 -> Out1/1

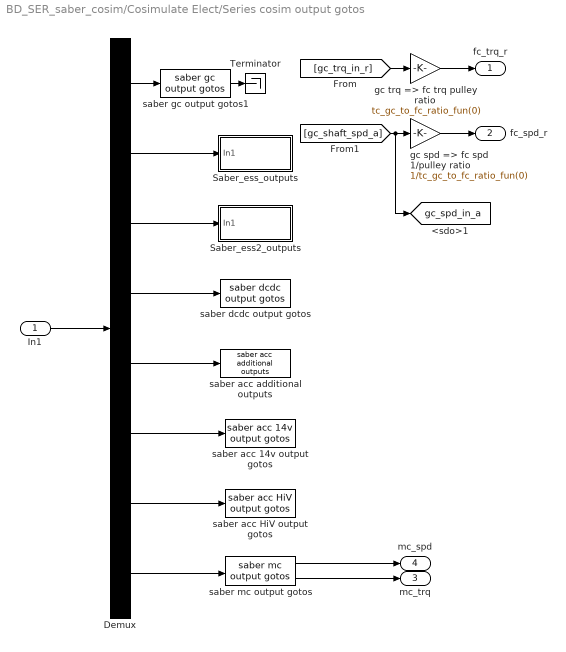
== system BD_SER_saber_cosim/Cosimulate Elect/Series cosim output gotos ==
  In1 : Inport  Port=1  LatchInput=off
  Demux : Demux  Outputs=[4 4 4 2 2 30 12 4]  BusSelectionMode=off
  Saber_ess2_outputs : Subsystem  BlockChoice=Saber_pb2
      settings: AttributesFormatString=%<BlockChoice>  TemplateBlock=lib_outputs/Saber_ess2_outputs  MemberBlocks=Saber_pb2,Saber_rint2  RTWFcnNameOpts=Auto  RTWFileNameOpts=Auto
  Saber_ess_outputs : Subsystem  BlockChoice=Saber_rint
      settings: AttributesFormatString=%<BlockChoice>  TemplateBlock=lib_outputs/Saber_ess_outputs  MemberBlocks=Saber_pb,Saber_rint  RTWFcnNameOpts=Auto  RTWFileNameOpts=Auto
  Terminator : Terminator
  gc spd => fc spd 1/pulley ratio : Gain  Gain=1/tc_gc_to_fc_ratio_fun(0)  Multiplication=Element-wise(K.*u)  SaturateOnIntegerOverflow=on
  gc trq => fc trq pulley ratio : Gain  Gain=tc_gc_to_fc_ratio_fun(0)  Multiplication=Element-wise(K.*u)  SaturateOnIntegerOverflow=on
  saber acc 14v output gotos : lib_outputs/saber acc 14v output gotos
      settings: RTWFcnNameOpts=Auto  RTWFileNameOpts=Auto
  saber acc HiV output gotos : lib_outputs/saber acc HiV output gotos
      settings: RTWFcnNameOpts=Auto  RTWFileNameOpts=Auto
  saber acc additional outputs : lib_outputs/saber acc additional outputs
      settings: RTWFcnNameOpts=Auto  RTWFileNameOpts=Auto
  saber dcdc output gotos : lib_outputs/saber dcdc output gotos
      settings: RTWFcnNameOpts=Auto  RTWFileNameOpts=Auto
  saber gc output gotos1 : lib_outputs/saber gc output gotos
      settings: RTWFcnNameOpts=Auto  RTWFileNameOpts=Auto
  saber mc output gotos : lib_outputs/saber mc output gotos
      link override sign convention: Gain=1
      settings: RTWFcnNameOpts=Auto  RTWFileNameOpts=Auto
  fc_trq_r : Outport  Port=1
  fc_spd_r : Outport  Port=2
  mc_trq : Outport  Port=3
  mc_spd : Outport  Port=4
  tag scope: gc_spd_in_a=global
  wires:
  Demux/3 -> Saber_ess2_outputs/1(In1)
  Demux/2 -> Saber_ess_outputs/1(In1)
  saber mc output gotos/1 -> mc_spd/1
  saber mc output gotos/2 -> mc_trq/1
  In1/1 -> Demux/1
  Demux/1 -> saber gc output gotos1/1
  [gc_trq_in_r] -> gc trq => fc trq pulley ratio/1
  [gc_shaft_spd_a] -> gc spd => fc spd 1/pulley ratio/1, [gc_spd_in_a]
  saber gc output gotos1/1 -> Terminator/1
  Demux/4 -> saber dcdc output gotos/1
  gc spd => fc spd 1/pulley ratio/1 -> fc_spd_r/1
  gc trq => fc trq pulley ratio/1 -> fc_trq_r/1
  Demux/6 -> saber acc 14v output gotos/1
  Demux/7 -> saber acc HiV output gotos/1
  Demux/8 -> saber mc output gotos/1
  Demux/5 -> saber acc additional outputs/1

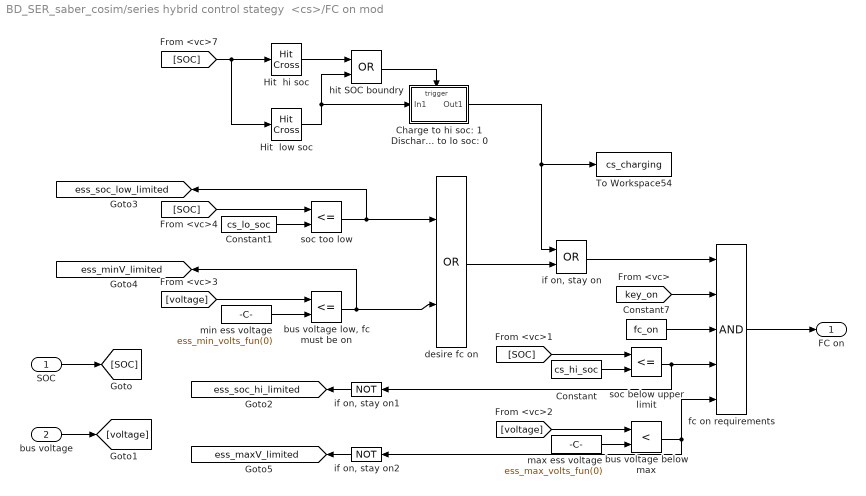
== system BD_SER_saber_cosim/series hybrid control stategy  <cs>/FC on mod ==
  SOC : Inport  Port=1  LatchInput=off  PortDimensions=1
  bus voltage : Inport  Port=2  LatchInput=off
  Charge to hi soc: 1 Discharge to lo soc: 0 : Subsystem  TreatAsAtomicUnit=on
      settings: RTWFcnNameOpts=Auto  RTWFileNameOpts=Auto
  Constant : Constant  Value=cs_hi_soc
  Constant1 : Constant  Value=cs_lo_soc
  Constant7 : Constant  Value=fc_on
  Hit  hi soc : HitCross  HitCrossingOffset=cs_hi_soc  HitCrossingDirection=rising  ShowOutputPort=on
  Hit  low soc : HitCross  HitCrossingOffset=cs_lo_soc  HitCrossingDirection=falling  ShowOutputPort=on
  To Workspace54 : ToWorkspace  VariableName=cs_charging  SampleTime=-1  SaveFormat=Array
  "bus voltage below max " : RelationalOperator  Operator=<
  "bus voltage low, fc must be on" : RelationalOperator  Operator=<=
  desire fc on : Logic  Operator=OR  Inputs=2
  fc on requirements : Logic  Operator=AND  Inputs=5
  hit SOC boundry : Logic  Operator=OR  Inputs=2
  "if on, stay on" : Logic  Operator=OR  Inputs=2
  "if on, stay on1" : Logic  Orientation=left  Operator=NOT  Inputs=2
  "if on, stay on2" : Logic  Orientation=left  Operator=NOT  Inputs=2
  max ess voltage : Constant  Value=ess_max_volts_fun(0)
  min ess voltage : Constant  Value=ess_min_volts_fun(0)
  soc below upper limit : RelationalOperator  Operator=<=
  soc too low : RelationalOperator  Operator=<=
  FC on : Outport  Port=1
  tag scope: ess_maxV_limited=global, ess_minV_limited=global, ess_soc_hi_limited=global, ess_soc_low_limited=global
  wires:
  Constant7/1 -> fc on requirements/3
  Constant/1 -> soc below upper limit/2
  min ess voltage/1 -> "bus voltage low, fc must be on"/2
  Constant1/1 -> soc too low/2
  max ess voltage/1 -> "bus voltage below max "/2
  SOC/1 -> [SOC]
  bus voltage/1 -> [voltage]
  [SOC] -> soc below upper limit/1
  [voltage] -> "bus voltage below max "/1
  [voltage] -> "bus voltage low, fc must be on"/1
  [SOC] -> soc too low/1
  fc on requirements/1 -> FC on/1
  [key_on] -> fc on requirements/2
  desire fc on/1 -> "if on, stay on"/2
  soc below upper limit/1 -> "if on, stay on1"/1, fc on requirements/4
  "bus voltage below max "/1 -> "if on, stay on2"/1, fc on requirements/5
  soc too low/1 -> desire fc on/1, [ess_soc_low_limited]
  "bus voltage low, fc must be on"/1 -> desire fc on/2, [ess_minV_limited]
  "if on, stay on"/1 -> fc on requirements/1
  Charge to hi soc: 1 Discharge to lo soc: 0/1(Out1) -> "if on, stay on"/1, To Workspace54/1
  hit SOC boundry/1 -> Charge to hi soc: 1 Discharge to lo soc: 0/Trigger
  Hit  hi soc/1 -> hit SOC boundry/1
  Hit  low soc/1 -> hit SOC boundry/2, Charge to hi soc: 1 Discharge to lo soc: 0/1(In1)
  [SOC] -> Hit  hi soc/1, Hit  low soc/1
  "if on, stay on1"/1 -> [ess_soc_hi_limited]
  "if on, stay on2"/1 -> [ess_maxV_limited]

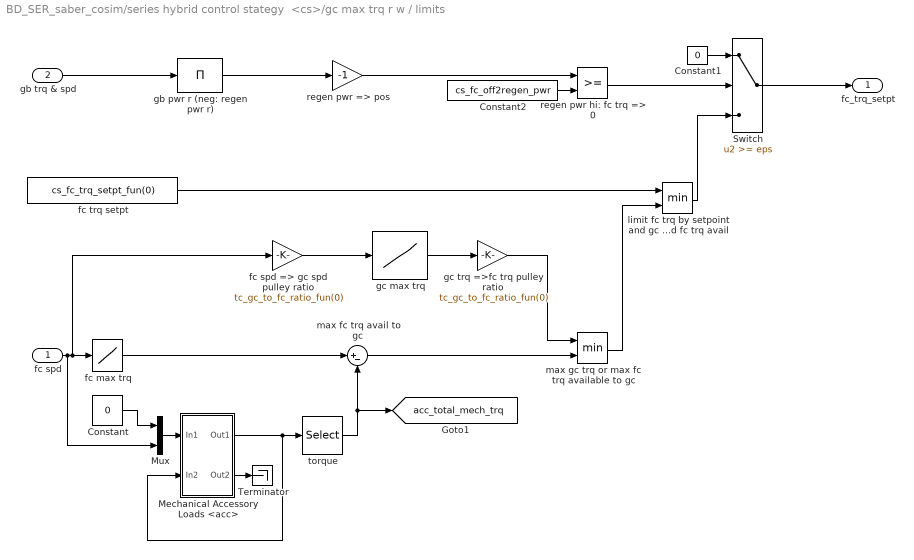
== system BD_SER_saber_cosim/series hybrid control stategy  <cs>/gc max trq r w / limits ==
  fc spd : Inport  Port=1  LatchInput=off
  gb trq & spd : Inport  Port=2  LatchInput=off
  Constant : Constant  Value=0
  Constant1 : Constant  Value=0
  Constant2 : Constant  Value=cs_fc_off2regen_pwr
  Mechanical Accessory Loads <acc> : Subsystem
      settings: RTWFcnNameOpts=Auto  RTWFileNameOpts=Auto
      mask Display: image(imread('bdi_acc_pic.bmp'))
  Mux : Mux  Inputs=2
  Switch : Switch  Threshold=eps
  Terminator : Terminator
  fc max trq : Lookup  InputValues=fc_map_spd*fc_spd_scale  OutputValues=fc_max_trq*fc_trq_scale
  fc spd => gc spd pulley ratio : Gain  Gain=tc_gc_to_fc_ratio_fun(0)  Multiplication=Element-wise(K.*u)  SaturateOnIntegerOverflow=on
  fc trq setpt : Constant  Value=cs_fc_trq_setpt_fun(0)
  gb pwr r (neg: regen pwr r) : Product  Inputs=1  Multiplication=Element-wise(.*)  SaturateOnIntegerOverflow=on
  gc max trq : Lookup  InputValues=gc_map_spd*gc_spd_scale  OutputValues=gc_max_trq*gc_trq_scale
  gc trq =>fc trq pulley ratio : Gain  Gain=tc_gc_to_fc_ratio_fun(0)  Multiplication=Element-wise(K.*u)  SaturateOnIntegerOverflow=on
  limit fc trq by setpoint and gc and fc trq avail : MinMax  Function=min  Inputs=2
  max fc trq avail to gc : Sum  Inputs=|+-  SaturateOnIntegerOverflow=on
  max gc trq or max fc trq available to gc : MinMax  Function=min  Inputs=2
  regen pwr => pos : Gain  Gain=-1  Multiplication=Element-wise(K.*u)  SaturateOnIntegerOverflow=on
  regen pwr hi: fc trq => 0 : RelationalOperator  Operator=>=
  torque : Selector  InputType=Vector  ElementSrc=Internal  Elements=1  RowSrc=Internal  Rows=1  ColumnSrc=Internal  Columns=1  InputPortWidth=2
  fc_trq_setpt : Outport  Port=1
  tag scope: acc_total_mech_trq=global
  wires:
  fc trq setpt/1 -> limit fc trq by setpoint and gc and fc trq avail/1
  fc spd/1 -> Mux/2, fc max trq/1, fc spd => gc spd pulley ratio/1
  fc max trq/1 -> max fc trq avail to gc/1
  max fc trq avail to gc/1 -> max gc trq or max fc trq available to gc/2
  Mux/1 -> Mechanical Accessory Loads <acc>/1(In1)
  Mechanical Accessory Loads <acc>/1(Out1) -> torque/1, Mechanical Accessory Loads <acc>/2(In2)
  torque/1 -> max fc trq avail to gc/2, [acc_total_mech_trq]
  Mechanical Accessory Loads <acc>/2(Out2) -> Terminator/1
  max gc trq or max fc trq available to gc/1 -> limit fc trq by setpoint and gc and fc trq avail/2
  gc max trq/1 -> gc trq =>fc trq pulley ratio/1
  fc spd => gc spd pulley ratio/1 -> gc max trq/1
  gc trq =>fc trq pulley ratio/1 -> max gc trq or max fc trq available to gc/1
  Constant/1 -> Mux/1
  Switch/1 -> fc_trq_setpt/1
  limit fc trq by setpoint and gc and fc trq avail/1 -> Switch/3
  Constant1/1 -> Switch/1
  Constant2/1 -> regen pwr hi: fc trq => 0/2
  gb pwr r (neg: regen pwr r)/1 -> regen pwr => pos/1
  regen pwr => pos/1 -> regen pwr hi: fc trq => 0/1
  regen pwr hi: fc trq => 0/1 -> Switch/2
  gb trq & spd/1 -> gb pwr r (neg: regen pwr r)/1

== system BD_SER_saber_cosim/<vc> series/gearbox control for series  HV and EV/Block NOTES ==
  note: This gearbox control block computes the current gear number given the gearbox's
      | req'd output torque and speed and an estimate its efficiency.  Upshifts occur, given a
      | certain engine speed,  when the estimated engine load falls below the upshift curve
      | in engine speed/load space, and downshifts likewise occur when estimated engine
      | load rises above the downshift curve.  Separate upshift and downshift curves are
      | defined for each gear.  An upshift may not be immediately followed by a downshift.
      | If the tires are about to slip, don't upshift unless the engine would be at max. speed.
      | Enforce this rule by setting the load to 1 when the tires are about to slip.

== system BD_SER_saber_cosim/<vc> series/gearbox control for series  HV and EV/allow downshift? ==
  prev gearnum : Inport  Port=1  LatchInput=off
  Logical Operator : Logic  Operator=NOR  Inputs=2
  Memory : Memory  X0=1  InheritSampleTime=off
      settings: RTWStateStorageClass=Auto
  Memory1 : Memory  X0=1  InheritSampleTime=off
      settings: RTWStateStorageClass=Auto
  Relational Operator1 : RelationalOperator  Operator=>
  Relational Operator2 : RelationalOperator  Operator=>
  allow shift : Outport  Port=1  InitialOutput=0
  wires:
  Relational Operator2/1 -> Logical Operator/2
  Memory1/1 -> Relational Operator2/2
  Memory/1 -> Memory1/1, Relational Operator1/2
  Relational Operator1/1 -> Logical Operator/1
  prev gearnum/1 -> Relational Operator2/1, Memory/1, Relational Operator1/1
  Logical Operator/1 -> allow shift/1

== system BD_SER_saber_cosim/<vc> series/gearbox control for series  HV and EV/downshift  command ==
  prev gear number : Inport  Port=1  LatchInput=off
  engine load : Inport  Port=2  LatchInput=off
  engine speed : Inport  Port=3  LatchInput=off
  Mux : Mux  Inputs=2
      settings: DisplayOption=none
  Relational Operator : RelationalOperator  Operator=>
  load fraction : Subsystem  mask(Gear Selector){spd=gb_dnshift_spd, load=gb_dnshift_load}
      mask prompts: spd "Speeds:"; load "Load Fractions:"
      mask help:
      | This block will perform a linear interplation (extrapolation outside of bounds) to determine the shift point load fraction associated with the current gear number and speed.
      |
      | The Speeds parameter should be defined as an array of vectors containing speeds for each gear number.  The Load Fractions parameter should be defined as a array of vectors containing load fractions indexed by the speeds in the Speeds parameter for each gear number.
      settings: RTWFcnNameOpts=Auto  RTWFileNameOpts=Auto
      mask Help:
      | Reference the base workspace variables - gb_**shift_spd and gb_**shift_load  where ** is either up for upshift conditions or dn for downshift conditions.
      | 
      | Or define the arrays as follows:
      | 
      | {[spd1 spd2 spd3 spd4]; [spd1 spd2 spd3 spd4]; ...}
      | 
      | {[load1 load2 load3 load4]; [load1 load2 load3 load4]; ...}
      | 
      | where each array contains one row for each gear in the gearbox.  Speeds should be defined in rad/s and loads as a decimal fraction.
  command : Outport  Port=1  InitialOutput=0
  wires:
  Relational Operator/1 -> command/1
  engine speed/1 -> Mux/2
  prev gear number/1 -> Mux/1
  engine load/1 -> Relational Operator/1
  Mux/1 -> load fraction/1(In1)
  load fraction/1(Out1) -> Relational Operator/2

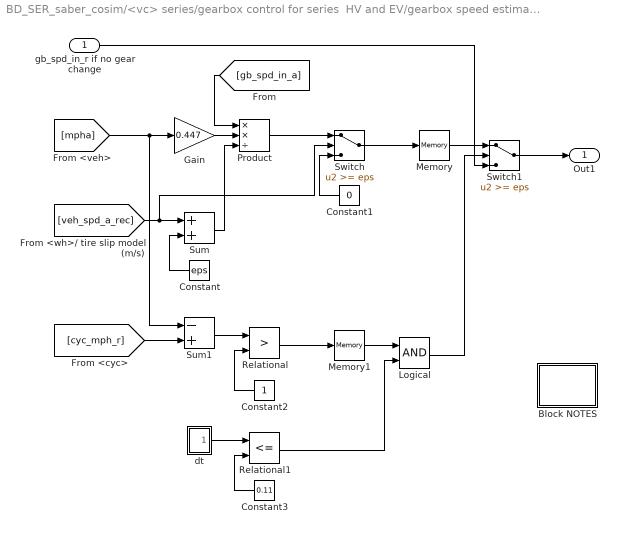
== system BD_SER_saber_cosim/<vc> series/gearbox control for series  HV and EV/gearbox speed estimator ==
  gb_spd_in_r if no gear change : Inport  Port=1  LatchInput=off
  Block NOTES : Subsystem
      settings: RTWFcnNameOpts=Auto  RTWFileNameOpts=Auto
      mask Display: disp('Block\nNOTES')
  Constant : Constant  Orientation=left  Value=eps
  Constant1 : Constant  Orientation=left  Value=0
  Constant2 : Constant  Orientation=left  Value=1
  Constant3 : Constant  Orientation=left  Value=0.11
  Gain : Gain  Gain=0.447  Multiplication=Element-wise(K.*u)  SaturateOnIntegerOverflow=on
  Logical : Logic  Operator=AND  Inputs=2
  Memory : Memory  X0=cyc_mph(1,2)*0.447/wh_radius*fd_ratio*gb_ratio(gb_num_init)  InheritSampleTime=off
      settings: RTWStateStorageClass=Auto
  Memory1 : Memory  X0=1  InheritSampleTime=off
      settings: RTWStateStorageClass=Auto
  Product : Product  Inputs=**/  Multiplication=Element-wise(.*)  SaturateOnIntegerOverflow=on
  Relational : RelationalOperator  Operator=>
  Relational1 : RelationalOperator  Operator=<=
  Sum : Sum  Inputs=++  SaturateOnIntegerOverflow=on
  Sum1 : Sum  Inputs=-+  SaturateOnIntegerOverflow=on
  Switch : Switch  Threshold=eps
  Switch1 : Switch  Threshold=eps
  dt : Subsystem
      settings: RTWFcnNameOpts=Auto  RTWFileNameOpts=Auto
  Out1 : Outport  Port=1
  wires:
  Constant3/1 -> Relational1/2
  Relational1/1 -> Logical/2
  Logical/1 -> Switch1/2
  Memory1/1 -> Logical/1
  dt/1(Out1) -> Relational1/1
  [gb_spd_in_a] -> Product/1
  gb_spd_in_r if no gear change/1 -> Switch1/3
  Switch1/1 -> Out1/1
  Switch/1 -> Memory/1
  Relational/1 -> Memory1/1
  Sum1/1 -> Relational/1
  Constant2/1 -> Relational/2
  [mpha] -> Sum1/1, Gain/1
  [cyc_mph_r] -> Sum1/2
  Constant/1 -> Sum/2
  Memory/1 -> Switch1/1
  Constant1/1 -> Switch/3
  [veh_spd_a_rec] -> Switch/2, Sum/1
  Gain/1 -> Product/2
  Sum/1 -> Product/3
  Product/1 -> Switch/1

== system BD_SER_saber_cosim/<vc> series/gearbox control for series  HV and EV/shifting1 ==
  gear number : Inport  Port=1  LatchInput=off
  Constant : Constant  Value=gb_shift_delay-1e-6
  Relational Operator : RelationalOperator  Operator=<
  time since last shift : Subsystem
      settings: RTWFcnNameOpts=Auto  RTWFileNameOpts=Auto
      mask Display: disp('time since\nlast shift')
  out_1 : Outport  Port=1  InitialOutput=0
  wires:
  time since last shift/1(out_1) -> Relational Operator/1
  Constant/1 -> Relational Operator/2
  gear number/1 -> time since last shift/1(in_1)
  Relational Operator/1 -> out_1/1

== system BD_SER_saber_cosim/<vc> series/gearbox control for series  HV and EV/upshift  command ==
  prev gear number : Inport  Port=1  LatchInput=off
  engine load : Inport  Port=2  LatchInput=off
  engine speed : Inport  Port=3  LatchInput=off
  Mux : Mux  Inputs=2
      settings: DisplayOption=none
  Relational Operator : RelationalOperator  Operator=<
  load fraction : Subsystem  mask(Gear Selector){spd=gb_upshift_spd, load=gb_upshift_load}
      mask prompts: spd "Speeds:"; load "Load Fractions:"
      mask help:
      | This block will perform a linear interplation (extrapolation outside of bounds) to determine the shift point load fraction associated with the current gear number and speed.
      |
      | The Speeds parameter should be defined as an array of vectors containing speeds for each gear number.  The Load Fractions parameter should be defined as a array of vectors containing load fractions indexed by the speeds in the Speeds parameter for each gear number.
      settings: RTWFcnNameOpts=Auto  RTWFileNameOpts=Auto
      mask Help:
      | Reference the base workspace variables - gb_**shift_spd and gb_**shift_load  where ** is either up for upshift conditions or dn for downshift conditions.
      | 
      | Or define the arrays as follows:
      | 
      | {[spd1 spd2 spd3 spd4]; [spd1 spd2 spd3 spd4]; ...}
      | 
      | {[load1 load2 load3 load4]; [load1 load2 load3 load4]; ...}
      | 
      | where each array contains one row for each gear in the gearbox.  Speeds should be defined in rad/s and loads as a decimal fraction.
  command : Outport  Port=1  InitialOutput=0
  wires:
  Relational Operator/1 -> command/1
  engine speed/1 -> Mux/2
  Mux/1 -> load fraction/1(In1)
  prev gear number/1 -> Mux/1
  engine load/1 -> Relational Operator/1
  load fraction/1(Out1) -> Relational Operator/2

== system BD_SER_saber_cosim/<vc> series/series 'clutch' control/Block NOTES ==
  note: There is no clutch, per se, in the series hybrid vehicle, that is connected to
      | the engine.  This clutch control is provided to tell the fuel converter (a.k.a. engine)
      | when it can spin up freely.  The fuel converter spins up or down when the 'clutch' is
      | disengaged, and provides torque when the 'clutch' is engaged (signal==3).
      |
      | Here, the fuel converter spins up when the engine has been off within the
      | past 0.5 s (or one time step, whichever is greater).  At all other times, the fuel
      | converter provides torque to the generator.

== system BD_SER_saber_cosim/Cosimulate Elect/Generator RPM Ach/Enabled Subsystem ==
  In1 : Inport  Port=1  LatchInput=off
  Enable : EnablePort
  Out1 : Outport  Port=1  InitialOutput=0
  wires:
  In1/1 -> Out1/1

== system BD_SER_saber_cosim/Cosimulate Elect/Model Data In/Aux Loads 14V and 42V ==
  Aux Loads 14V : lib_cosimulation/Aux Loads 14V
      settings: RTWFcnNameOpts=Auto  RTWFileNameOpts=Auto
  Aux Loads 42V : lib_cosimulation/Aux Loads 42V
      settings: RTWFcnNameOpts=Auto  RTWFileNameOpts=Auto
  Elec Aux Loads Additional : lib_cosimulation/Elec Aux Loads Additional
      settings: RTWFcnNameOpts=Auto  RTWFileNameOpts=Auto
  Matrix Concatenation1 : S-Function  FunctionName=smatrxcat  Parameters=numInports,catMethod  PortCounts=[]  SFunctionModules=''  mask(Matrix Concatenation){numInports=3, catMethod=Horizontal}
      mask prompts: numInports "Number of inputs:"; catMethod "Concatenation method:"
      mask help: Perform horizontal or vertical concatenation. 1-D vector input signals are treated as column vectors, i.e., [Mx1] matrices. The output is always a matrix.
      mask init:
      | xy = matrxcatmask('icon');
      mask StyleString: edit,popup(Horizontal|Vertical)
      mask Display:
      | plot(xy.x,xy.y);
      | text(0.15,0.86,xy.label);
  Out1 : Outport  Port=1
  wires:
  Matrix Concatenation1/1 -> Out1/1
  Aux Loads 42V/1 -> Matrix Concatenation1/3
  Aux Loads 14V/1 -> Matrix Concatenation1/2
  Elec Aux Loads Additional/1 -> Matrix Concatenation1/1

== system BD_SER_saber_cosim/Cosimulate Elect/Model Data In/ess param inputs ==
  Rint : lib_cosimulation/Rint
      settings: RTWFcnNameOpts=Auto  RTWFileNameOpts=Auto
  Out1 : Outport  Port=1
  wires:
  Rint/1 -> Out1/1

== system BD_SER_saber_cosim/Cosimulate Elect/Model Data In/ess2 param inputs ==
  Saber lib pb2 : lib_cosimulation/Saber lib pb2
      settings: RTWFcnNameOpts=Auto  RTWFileNameOpts=Auto
  Out1 : Outport  Port=1
  wires:
  Saber lib pb2/1 -> Out1/1
